simulink model "MPC_Controller"  (Simulink 9.1)
settings: Solver=ode45  StartTime=0  StopTime=6  FixedStep=TSTEP  RelTol=1e-3  EnableMultiTasking=on
PreLoadFcn:
  | cd extensions\simulink\pt_center_diff
  | Run_ft4wd_eclass
  | lsd_parameta_eclass
  | cd ..\..\..
libraries: Solver_SF x1, simulink x1
settings Model: Creator=ywata  LastModifiedBy=小Y  ExtModeTrigMode=oneshot  ExtModeArmWhenConnect=off
settings SolverCC: AlgebraicLoopSolver=LineSearch
settings DataIOCC: SignalLoggingSaveFormat=ModelDataLogs  SaveOutput=off  SaveTime=off  SignalLoggingName=sigsOut
settings OptimizationCC: BooleanDataType=off
settings DebuggingCC: SaveWithParameterizedLinksMsg=none  SignalResolutionControl=TryResolveAllWithWarning  MultiTaskDSMMsg=warning  MultiTaskCondExecSysMsg=none  FcnCallInpInsideContextMsg=warning  StateNameClashWarn=warning
settings HardwareCC: TargetBitPerPointer=64  TargetBitPerSizeT=64  TargetBitPerPtrDiffT=64  TargetLongLongMode=on  TargetIntDivRoundTo=Zero  TargetEndianess=LittleEndian  TargetWordSize=64  TargetHWDeviceType=MATLAB Host  ProdEqTarget=off
settings GRTTargetCC: TargetFcnLib=ansi_tfl_tmw.mat  ModelReferenceCompliant=off  MatFileLogging=off

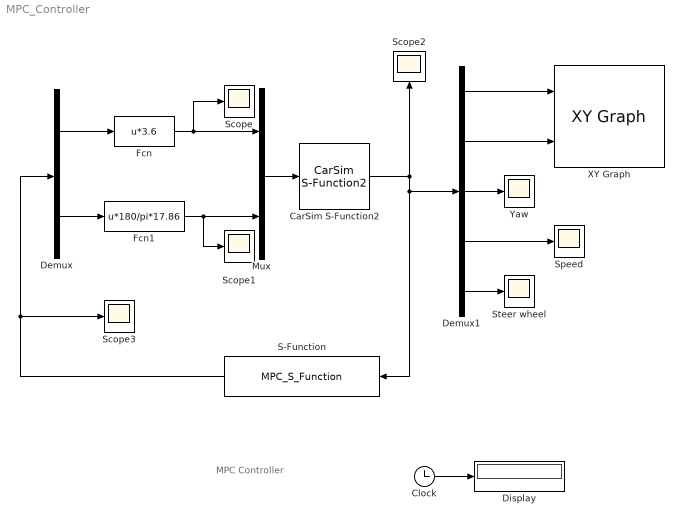
== system MPC_Controller ==
  note: MPC Controller
  CarSim S-Function2 : Solver_SF/CarSim S-Function2  Priority=1  VehicleCode=i_s  SIMFILE=simfile.sim
      settings: AttributesFormatString=Vehicle Code: %<VehicleCode>
  Clock : Clock
  Demux : Demux  Outputs=2
  Demux1 : Demux  Outputs=5
  Display : Display
  Fcn : Fcn  Expr=u*3.6
  Fcn1 : Fcn  Expr=u*180/pi*17.86
  Mux : Mux  Inputs=2
  S-Function : S-Function  FunctionName=MPC_S_Function  SFunctionDeploymentMode=off  EnableBusSupport=off
  Scope{,1..3} (4 alike) : Scope
  Speed : Scope
  Steer wheel : Scope
  XY Graph : simulink/Sinks/XY Graph  xmin=-1  xmax=100  ymin=-5  ymax=5  st=-1
  Yaw : Scope
  wires:
  Clock/1 -> Display/1
  Mux/1 -> CarSim S-Function2/1
  Demux1/4 -> Speed/1
  Demux1/3 -> Yaw/1
  Demux1/2 -> XY Graph/2
  Demux1/1 -> XY Graph/1
  Demux1/5 -> Steer wheel/1
  S-Function/1 -> Demux/1, Scope3/1
  Fcn/1 -> Mux/1, Scope/1
  Fcn1/1 -> Mux/2, Scope1/1
  CarSim S-Function2/1 -> Demux1/1, S-Function/1, Scope2/1
  Demux/1 -> Fcn/1
  Demux/2 -> Fcn1/1
